simulink model "playback"  (R2016b)
settings: Solver=FixedStepDiscrete  StartTime=47  StopTime=49  FixedStep=sample_time  RelTol=1e-3
undefined symbols (not defined in the file or in its folder): A_kalman_sea_swing, A_lpf_dtau, B1_lpf_dtau, B2_lpf_dtau, B_kalman_sea_swing, C_kalman_sea_swing, control_start_time, Discrete, fdesignblkfcn, gcbh, initial_dx_estimate, k_sea_low, kalman_load_to_deflect_transmission, lateral_motor_efficiency, P0_kalman_sea_swing, Q_kalman_rotor_torque, Q_kalman_spring_torque, Q_kalman_trunk_torque, R_kalman_absolute_fail, R_kalman_absolute_normal, R_kalman_incremental_loaded, R_kalman_incremental_unloaded, sample_time, Time
libraries: simulink x4, ctrlSharedLib x4, dsparch4 x1
settings Model: Creator=wmartin  LastModifiedBy=Will
settings SolverCC: EnableConcurrentExecution=on
settings DataIOCC: MaxDataPoints=1000000000  SaveFormat=StructureWithTime  SignalLogging=off  DSMLogging=off  VisualizeSimOutput=off
settings OptimizationCC: BlockReduction=off  OptimizeBlockIOStorage=off  BufferReuse=off  GlobalBufferReuse=off  ExpressionFolding=off  ExpressionDepthLimit=2147483647  LocalBlockOutputs=off  LifeSpan=inf  SimCompilerOptimization=on
settings DebuggingCC: UnderspecifiedInitializationDetection=Classic  MergeDetectMultiDrivingBlocksExec=none  SolverPrmCheckMsg=warning  StateNameClashWarn=warning  SFUnexpectedBacktrackingDiag=warning  SFNoUnconditionalDefaultTransitionDiag=warning  SFExecutionAtInitializationDiag=none
settings HardwareCC: ProdBitPerPointer=32  ProdBitPerSizeT=32  ProdBitPerPtrDiffT=32  ProdLargestAtomicFloat=None  ProdWordSize=32  ProdLongLongMode=on  ProdHWDeviceType=Generic->32-bit x86 compatible
settings ModelReferenceCC: UpdateModelReferenceTargets=IfOutOfDate  ModelReferenceNumInstancesAllowed=Single  ModelReferenceMinAlgLoopOccurrences=on  PropagateSignalLabelsOutOfModel=off
settings RTWCC: SystemTargetFile=slrt.tlc  TemplateMakefile=slrt_default_tmf  Description=Simulink Real-Time  RTWVerbose=off  RTWCompilerOptimization=on
settings CodeAppCC: MaxIdLength=256
settings SimulinkRealTimeCC: GeneratePreprocessorConditionals=Disable all
settings ConfigComp: CovMetricSettings=dw  CovHtmlReporting=on  CovSaveCumulativeToWorkspaceVar=on  CovSaveSingleToWorkspaceVar=on  CovExternalEMLEnable=off  CovSFcnEnable=off

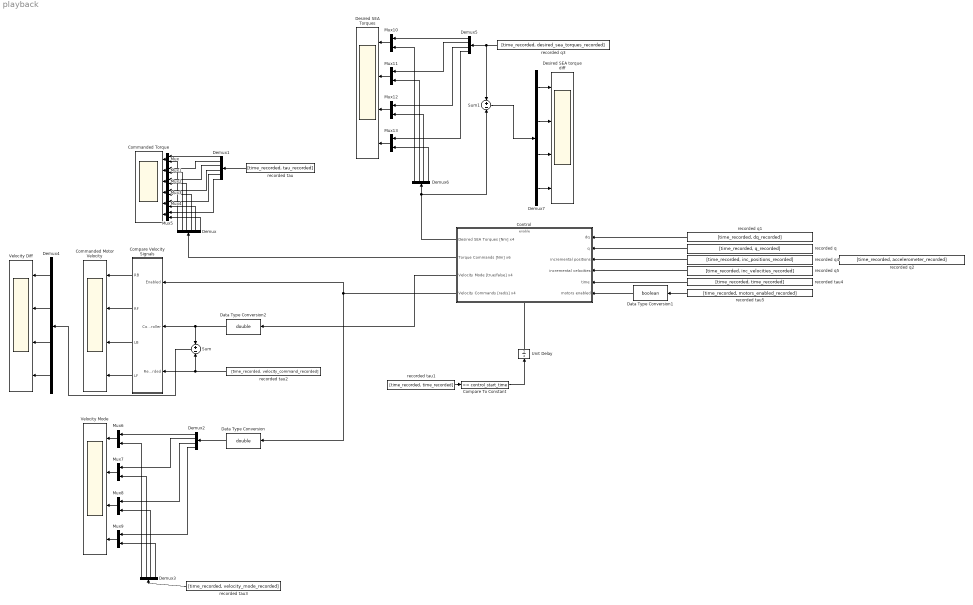
== system playback ==
  Commanded Motor Velocity : Scope  NumInputPorts=4
  Commanded Torque : Scope  NumInputPorts=6
  Compare To Constant : simulink/Logic and Bit Operations/Compare To Constant  relop=>=  const=control_start_time  OutDataTypeStr=boolean
  Compare Velocity Signals : Subsystem
  Control : Subsystem
  Data Type Conversion : DataTypeConversion  OutDataTypeStr=double
  Data Type Conversion1 : DataTypeConversion  OutDataTypeStr=boolean
  Data Type Conversion2 : DataTypeConversion  OutDataTypeStr=double
  Demux : Demux  Outputs=6
  Demux1 : Demux  Outputs=6
  Demux{2..7} (6 alike) : Demux
  Desired SEA Torques : Scope  NumInputPorts=4
  Desired SEA torque diff : Scope  NumInputPorts=4
  Mux{,1..13} (14 alike) : Mux  Inputs=2
  Sum : Sum  Inputs=+-
  Sum1 : Sum  Inputs=+-
  Unit Delay : UnitDelay  SampleTime=-1
  Velocity Diff : Scope  NumInputPorts=4
  Velocity Mode : Scope  NumInputPorts=4
  recorded q : FromWorkspace  VariableName=[time_recorded, q_recorded]  OutDataTypeStr=double  SampleTime=sample_time  OutputAfterFinalValue=Holding final value
  recorded q1 : FromWorkspace  VariableName=[time_recorded, dq_recorded]  OutDataTypeStr=double  SampleTime=sample_time  OutputAfterFinalValue=Holding final value
  recorded q2 : FromWorkspace  VariableName=[time_recorded, accelerometer_recorded]  OutDataTypeStr=double  SampleTime=sample_time  OutputAfterFinalValue=Holding final value
  recorded q3 : FromWorkspace  VariableName=[time_recorded, desired_sea_torques_recorded]  OutDataTypeStr=double  SampleTime=sample_time  OutputAfterFinalValue=Holding final value
  recorded q4 : FromWorkspace  VariableName=[time_recorded, inc_positions_recorded]  OutDataTypeStr=double  SampleTime=sample_time  OutputAfterFinalValue=Holding final value
  recorded q5 : FromWorkspace  VariableName=[time_recorded, inc_velocities_recorded]  OutDataTypeStr=double  SampleTime=sample_time  OutputAfterFinalValue=Holding final value
  recorded tau : FromWorkspace  VariableName=[time_recorded, tau_recorded]  OutDataTypeStr=double  SampleTime=sample_time  Interpolate=off  OutputAfterFinalValue=Holding final value
  recorded tau1 : FromWorkspace  VariableName=[time_recorded, time_recorded]  OutDataTypeStr=double  SampleTime=sample_time  OutputAfterFinalValue=Holding final value
  recorded tau2 : FromWorkspace  VariableName=[time_recorded, velocity_command_recorded]  OutDataTypeStr=double  SampleTime=sample_time  Interpolate=off  OutputAfterFinalValue=Holding final value
  recorded tau3 : FromWorkspace  VariableName=[time_recorded, velocity_mode_recorded]  OutDataTypeStr=double  SampleTime=sample_time  Interpolate=off  OutputAfterFinalValue=Holding final value
  recorded tau4 : FromWorkspace  VariableName=[time_recorded, time_recorded]  OutDataTypeStr=double  SampleTime=sample_time  OutputAfterFinalValue=Holding final value
  recorded tau5 : FromWorkspace  VariableName=[time_recorded, motors_enabled_recorded]  OutDataTypeStr=double  SampleTime=sample_time  OutputAfterFinalValue=Holding final value
  wires:
  recorded tau1/1 -> Compare To Constant/1
  Compare To Constant/1 -> Unit Delay/1
  Unit Delay/1 -> Control/Enable
  Control/2(Torque Commands [Nm] x6) -> Demux/1
  recorded tau/1 -> Demux1/1
  Mux/1 -> Commanded Torque/1
  Mux1/1 -> Commanded Torque/2
  Mux2/1 -> Commanded Torque/3
  Mux3/1 -> Commanded Torque/4
  Mux4/1 -> Commanded Torque/5
  Mux5/1 -> Commanded Torque/6
  Demux1/1 -> Mux/1
  Demux/1 -> Mux/2
  Demux1/2 -> Mux1/1
  Demux1/3 -> Mux2/1
  Demux1/4 -> Mux3/1
  Demux1/5 -> Mux4/1
  Demux1/6 -> Mux5/1
  Demux/2 -> Mux1/2
  Demux/3 -> Mux2/2
  Demux/4 -> Mux3/2
  Demux/5 -> Mux4/2
  Demux/6 -> Mux5/2
  Compare Velocity Signals/1(RB) -> Commanded Motor Velocity/1
  Compare Velocity Signals/2(RF) -> Commanded Motor Velocity/2
  Compare Velocity Signals/3(LB) -> Commanded Motor Velocity/3
  Compare Velocity Signals/4(LF) -> Commanded Motor Velocity/4
  Control/4(Velocity Commands [rad/s] x4) -> Compare Velocity Signals/1(Enabled), Data Type Conversion/1
  recorded tau2/1 -> Sum/2, Compare Velocity Signals/3(Recorded)
  Mux6/1 -> Velocity Mode/1
  Mux7/1 -> Velocity Mode/2
  Mux8/1 -> Velocity Mode/3
  Mux9/1 -> Velocity Mode/4
  Demux2/2 -> Mux7/1
  Demux2/3 -> Mux8/1
  Demux2/4 -> Mux9/1
  recorded tau3/1 -> Demux3/1
  Demux3/1 -> Mux6/2
  Demux3/2 -> Mux7/2
  Demux3/3 -> Mux8/2
  Demux3/4 -> Mux9/2
  Data Type Conversion/1 -> Demux2/1
  Demux2/1 -> Mux6/1
  Control/3(Velocity Mode [true/false] x4) -> Data Type Conversion2/1
  Sum/1 -> Demux4/1
  Demux4/4 -> Velocity Diff/4
  Demux4/3 -> Velocity Diff/3
  Demux4/2 -> Velocity Diff/2
  Demux4/1 -> Velocity Diff/1
  Mux10/1 -> Desired SEA Torques/1
  Mux11/1 -> Desired SEA Torques/2
  Mux12/1 -> Desired SEA Torques/3
  Mux13/1 -> Desired SEA Torques/4
  Demux5/2 -> Mux11/1
  Demux5/3 -> Mux12/1
  Demux5/4 -> Mux13/1
  Demux6/1 -> Mux10/2
  Demux6/2 -> Mux11/2
  Demux6/3 -> Mux12/2
  Demux6/4 -> Mux13/2
  recorded q3/1 -> Demux5/1, Sum1/1
  Demux5/1 -> Mux10/1
  Control/1(Desired SEA Torques [Nm] x4) -> Sum1/2, Demux6/1
  Demux7/3 -> Desired SEA torque diff/3
  Demux7/2 -> Desired SEA torque diff/2
  Demux7/1 -> Desired SEA torque diff/1
  Demux7/4 -> Desired SEA torque diff/4
  Sum1/1 -> Demux7/1
  recorded q1/1 -> Control/1(dq)
  recorded q/1 -> Control/2(q)
  recorded tau4/1 -> Control/5(time)
  Data Type Conversion1/1 -> Control/6(motors enabled)
  recorded tau5/1 -> Data Type Conversion1/1
  recorded q4/1 -> Control/3(incremental positions)
  recorded q5/1 -> Control/4(incremental velocities)
  Data Type Conversion2/1 -> Sum/1, Compare Velocity Signals/2(Controller)

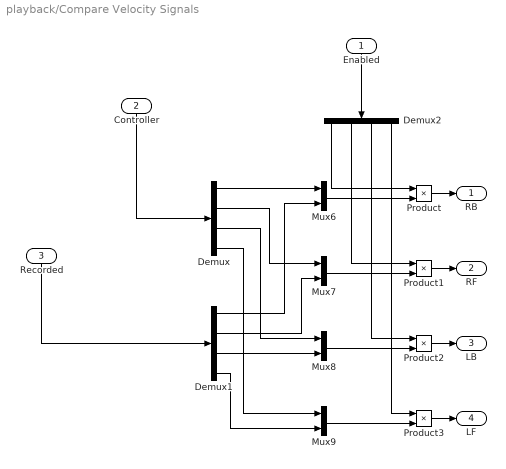
== system playback/Compare Velocity Signals ==
  Enabled : Inport
  Controller : Inport  Port=2
  Recorded : Inport  Port=3
  Demux : Demux
  Demux1 : Demux
  Demux2 : Demux
  Mux{6..9} (4 alike) : Mux  Inputs=2
  Product{,1..3} (4 alike) : Product
  RB : Outport
  RF : Outport  Port=2
  LB : Outport  Port=3
  LF : Outport  Port=4
  wires:
  Demux/3 -> Mux8/1
  Demux/2 -> Mux7/1
  Demux1/1 -> Mux6/2
  Demux/1 -> Mux6/1
  Product/1 -> RB/1
  Demux/4 -> Mux9/1
  Mux6/1 -> Product/2
  Demux1/4 -> Mux9/2
  Mux7/1 -> Product1/2
  Mux9/1 -> Product3/2
  Recorded/1 -> Demux1/1
  Demux2/3 -> Product2/1
  Demux1/2 -> Mux7/2
  Controller/1 -> Demux/1
  Demux2/1 -> Product/1
  Product3/1 -> LF/1
  Product1/1 -> RF/1
  Product2/1 -> LB/1
  Mux8/1 -> Product2/2
  Demux1/3 -> Mux8/2
  Enabled/1 -> Demux2/1
  Demux2/4 -> Product3/1
  Demux2/2 -> Product1/1

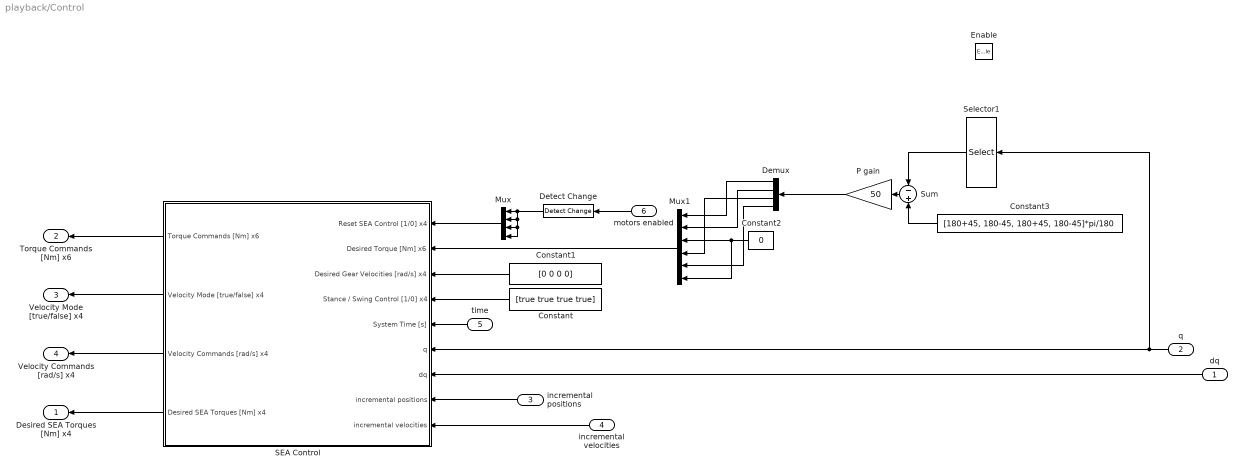
== system playback/Control ==
  dq : Inport
  q : Inport  Port=2
  incremental positions : Inport  Port=3
  incremental velocities : Inport  Port=4
  time : Inport  Port=5
  motors enabled : Inport  Port=6
  Enable : EnablePort  StatesWhenEnabling=reset  PropagateVarSize=During execution  ShowOutputPort=on
  Constant : Constant  Value=[true true true true]
  Constant1 : Constant  Value=[0 0 0 0]
  Constant2 : Constant  Value=0
  Constant3 : Constant  Value=[180+45, 180-45, 180+45, 180-45]*pi/180
  Demux : Demux
  Detect Change : simulink/Logic and Bit Operations/Detect Change  vinit=0  InputProcessing=Inherited  OutDataTypeStr=boolean
  Mux : Mux
  Mux1 : Mux  Inputs=6
  P gain : Gain  Gain=50
  SEA Control : Subsystem
  Selector1 : Selector  InputPortWidth=13  IndexOptions=Index vector (dialog)  Indices=[1 3 5 7]  OutputSizes=1
  Sum : Sum  Inputs=-+
  Desired SEA Torques [Nm] x4 : Outport  InitialOutput=[0 0 0 0]
  Torque Commands [Nm] x6 : Outport  Port=2  InitialOutput=[0 0 0 0 0 0]
  Velocity Mode [true/false] x4 : Outport  Port=3  InitialOutput=[false false false false]
  Velocity Commands [rad/s] x4 : Outport  Port=4  InitialOutput=[0 0 0 0]
  wires:
  incremental velocities/1 -> SEA Control/9(incremental velocities)
  incremental positions/1 -> SEA Control/8(incremental positions)
  P gain/1 -> Demux/1
  Sum/1 -> P gain/1
  Constant3/1 -> Sum/2
  Selector1/1 -> Sum/1
  Demux/4 -> Mux1/5
  Demux/3 -> Mux1/4
  Demux/2 -> Mux1/2
  Demux/1 -> Mux1/1
  Constant2/1 -> Mux1/3, Mux1/6
  SEA Control/4(Desired SEA Torques [Nm] x4) -> Desired SEA Torques [Nm] x4/1
  SEA Control/3(Velocity Commands [rad/s] x4) -> Velocity Commands [rad/s] x4/1
  SEA Control/2(Velocity Mode [true/false] x4) -> Velocity Mode [true/false] x4/1
  SEA Control/1(Torque Commands [Nm] x6) -> Torque Commands [Nm] x6/1
  Constant/1 -> SEA Control/4(Stance / Swing Control [1/0] x4)
  Constant1/1 -> SEA Control/3(Desired Gear Velocities [rad/s] x4)
  Mux1/1 -> SEA Control/2(Desired Torque [Nm] x6)
  Mux/1 -> SEA Control/1(Reset SEA Control [1/0] x4)
  dq/1 -> SEA Control/7(dq)
  q/1 -> Selector1/1, SEA Control/6(q)
  motors enabled/1 -> Detect Change/1
  Detect Change/1 -> Mux/4, Mux/3, Mux/2, Mux/1
  time/1 -> SEA Control/5(System Time [s])

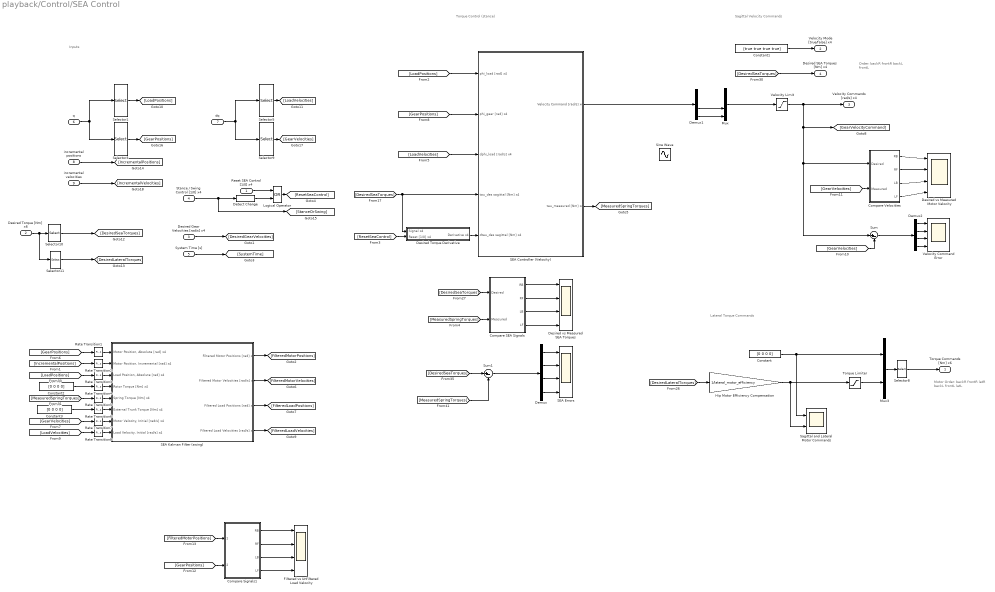
== system playback/Control/SEA Control ==
  note: Sagittal Velocity Commands
  note: Lateral Torque Commands
  note: Inputs
  note: Torque Control (stance)
  note: Motor Order:
      |
      | backR
      | frontR
      | latR
      | backL
      | frontL
      | latL
  note: Order:
      | backR
      | frontR
      | backL
      | frontL
  Reset SEA Control [1/0] x4 : Inport  OutDataTypeStr=boolean  PortDimensions=4  SampleTime=sample_time
  Desired Torque [Nm] x6 : Inport  Port=2  OutDataTypeStr=double  PortDimensions=6  SampleTime=sample_time
  Desired Gear Velocities [rad/s] x4 : Inport  Port=3  OutDataTypeStr=double  PortDimensions=4  SampleTime=sample_time
  Stance / Swing Control [1/0] x4 : Inport  Port=4  OutDataTypeStr=boolean  PortDimensions=4  SampleTime=sample_time
  System Time [s] : Inport  Port=5  OutDataTypeStr=double  PortDimensions=1  SampleTime=sample_time
  q : Inport  Port=6  OutDataTypeStr=double  PortDimensions=13  SampleTime=sample_time
  dq : Inport  Port=7  OutDataTypeStr=double  PortDimensions=13  SampleTime=sample_time
  incremental positions : Inport  Port=8  OutDataTypeStr=double  PortDimensions=4  SampleTime=sample_time
  incremental velocities : Inport  Port=9  OutDataTypeStr=double  PortDimensions=4  SampleTime=sample_time
  Compare SEA Signals : Subsystem
  Compare Signals1 : Subsystem
  Compare Velocities : Subsystem
  Constant : Constant  Value=[0 0 0 0]
  Constant1 : Constant  Value=[true true true true]
  Constant2 : Constant  Value=[0 0 0 0]
  Constant3 : Constant  Value=[0 0 0 0]
  Demux : Demux
  Demux1 : Demux
  Demux2 : Demux
  Desired Torque Derivative : Subsystem
  Desired vs Measured Motor Velocity : Scope  NumInputPorts=4
  Desired vs Measured SEA Torques : Scope  NumInputPorts=4
  Detect Change : simulink/Logic and Bit Operations/Detect Change  vinit=0  InputProcessing=Inherited  OutDataTypeStr=boolean
  Filtered vs Unfiltered Load Velocity : Scope  NumInputPorts=4
  Hip Motor Efficiency Compensation : Gain  Gain=1/lateral_motor_efficiency
  Logical Operator : Logic  Operator=OR  AllPortsSameDT=off  OutDataTypeStr=boolean
  Mux : Mux
  Mux3 : Mux  Inputs=2
  Rate Transition{1..8} (8 alike) : RateTransition  OutPortSampleTime=sample_time
  SEA Controller (Velocity) : Subsystem
  SEA Errors : Scope  NumInputPorts=4
  SEA Kalman Filter (swing) : Subsystem
  Sagittal and Lateral Motor Commands : Scope  NumInputPorts=2
  Selector1 : Selector  InputPortWidth=13  IndexOptions=Index vector (dialog)  Indices=[1 3 5 7]  OutputSizes=1
  Selector10 : Selector  InputPortWidth=6  IndexOptions=Index vector (dialog)  Indices=[1 2 4 5]  OutputSizes=1
  Selector11 : Selector  InputPortWidth=6  IndexOptions=Index vector (dialog)  Indices=[3 6]  OutputSizes=1
  Selector3 : Selector  InputPortWidth=13  IndexOptions=Index vector (dialog)  Indices=[2 4 6 8]  OutputSizes=1
  Selector5 : Selector  InputPortWidth=13  IndexOptions=Index vector (dialog)  Indices=[1 3 5 7]  OutputSizes=1
  Selector8 : Selector  InputPortWidth=6  IndexOptions=Index vector (dialog)  Indices=[1 2 5 3 4 6]  OutputSizes=1
  Selector9 : Selector  InputPortWidth=13  IndexOptions=Index vector (dialog)  Indices=[2 4 6 8]  OutputSizes=1
  Sine Wave : Sin  Amplitude=0.2  Frequency=68*2*pi  SampleTime=sample_time
  Sum : Sum  Inputs=|+-
  Sum1 : Sum  Inputs=|+-
  Torque Limiter : Saturate  UpperLimit=200  LowerLimit=-200
      settings: AttributesFormatString=Hi: %<UpperLimit>\nLo: %<LowerLimit>
  Velocity Command Error : Scope  NumInputPorts=4
  Velocity Limit : Saturate  UpperLimit=6  LowerLimit=-6
      settings: AttributesFormatString=Hi: %<UpperLimit>\nLo: %<LowerLimit>
  Torque Commands [Nm] x6 : Outport  OutDataTypeStr=double  PortDimensions=6  SampleTime=sample_time  InitialOutput=[0 0 0 0 0 0]
  Velocity Mode [true/false] x4 : Outport  Port=2  InitialOutput=[false false false false]
  Velocity Commands [rad/s] x4 : Outport  Port=3  InitialOutput=[0 0 0 0]
  Desired SEA Torques [Nm] x4 : Outport  Port=4  InitialOutput=[false false false false]
  wires:
  SEA Kalman Filter (swing)/4(Filtered Load Velocities [rad/s] x4) -> [FilteredLoadVelocities]
  SEA Kalman Filter (swing)/2(Filtered Motor Velocities [rad/s] x4) -> [FilteredMotorVelocities]
  SEA Kalman Filter (swing)/3(Filtered Load Positions [rad] x4) -> [FilteredLoadPositions]
  SEA Kalman Filter (swing)/1(Filtered Motor Positions [rad] x4) -> [FilteredMotorPositions]
  Constant3/1 -> Rate Transition6/1
  [LoadVelocities] -> Rate Transition8/1
  [GearVelocities] -> Rate Transition7/1
  Constant2/1 -> Rate Transition4/1
  [IncrementalPositions] -> Rate Transition2/1
  [GearPositions] -> Rate Transition1/1
  [LoadPositions] -> Rate Transition3/1
  [MeasuredSpringTorques] -> Rate Transition5/1
  incremental velocities/1 -> [IncrementalVelocities]
  incremental positions/1 -> [IncrementalPositions]
  Demux1/3 -> Mux/3
  Demux1/4 -> Mux/4
  Mux/1 -> Velocity Limit/1
  Torque Limiter/1 -> Mux3/2
  Sum1/1 -> Demux/1
  Demux/2 -> SEA Errors/2
  Demux/3 -> SEA Errors/3
  Demux/4 -> SEA Errors/4
  Demux/1 -> SEA Errors/1
  [DesiredSeaTorques] -> Sum1/1
  [MeasuredSpringTorques] -> Sum1/2
  Velocity Limit/1 -> Velocity Commands [rad/s] x4/1, Compare Velocities/1(Desired), Sum/1, [GearVelocityCommand]
  System Time [s]/1 -> [SystemTime]
  Selector9/1 -> [GearVelocities]
  Desired Gear Velocities [rad/s] x4/1 -> [DesiredGearVelocities]
  Detect Change/1 -> Logical Operator/2
  SEA Controller (Velocity)/1(Velocity Command [rad/s] x4) -> Demux1/1
  Selector10/1 -> [DesiredSeaTorques]
  Demux2/1 -> Velocity Command Error/1
  Demux2/2 -> Velocity Command Error/2
  Demux2/3 -> Velocity Command Error/3
  Demux2/4 -> Velocity Command Error/4
  Sum/1 -> Demux2/1
  [GearVelocities] -> Sum/2
  [GearVelocities] -> Compare Velocities/2(Measured)
  [GearPositions] -> SEA Controller (Velocity)/2(phi_gear [rad] x4)
  dq/1 -> Selector9/1, Selector5/1
  Selector3/1 -> [GearPositions]
  [LoadVelocities] -> SEA Controller (Velocity)/3(dphi_load [rad/s] x4)
  [DesiredSeaTorques] -> Desired SEA Torques [Nm] x4/1
  Reset SEA Control [1/0] x4/1 -> Logical Operator/1
  Logical Operator/1 -> [ResetSeaControl]
  Stance / Swing Control [1/0] x4/1 -> Detect Change/1, [StanceOrSwing]
  Constant1/1 -> Velocity Mode [true/false] x4/1
  [ResetSeaControl] -> Desired Torque Derivative/2(Reset [1/0] x4)
  [DesiredSeaTorques] -> Compare SEA Signals/1(Desired)
  Selector11/1 -> [DesiredLateralTorques]
  Desired Torque [Nm] x6/1 -> Selector10/1, Selector11/1
  Selector5/1 -> [LoadVelocities]
  Selector1/1 -> [LoadPositions]
  [MeasuredSpringTorques] -> Compare SEA Signals/2(Measured)
  Compare Velocities/2(RF) -> Desired vs Measured Motor Velocity/2
  Compare Velocities/1(RB) -> Desired vs Measured Motor Velocity/1
  Compare Velocities/3(LB) -> Desired vs Measured Motor Velocity/3
  Compare Velocities/4(LF) -> Desired vs Measured Motor Velocity/4
  Compare SEA Signals/4(LF) -> Desired vs Measured SEA Torques/4
  Compare SEA Signals/3(LB) -> Desired vs Measured SEA Torques/3
  Compare SEA Signals/2(RF) -> Desired vs Measured SEA Torques/2
  Compare SEA Signals/1(RB) -> Desired vs Measured SEA Torques/1
  Hip Motor Efficiency Compensation/1 -> Torque Limiter/1, Sagittal and Lateral Motor Commands/2
  Constant/1 -> Mux3/1, Sagittal and Lateral Motor Commands/1
  Desired Torque Derivative/1(Derivative x4) -> SEA Controller (Velocity)/5(dtau_des sagittal [Nm] x4)
  Mux3/1 -> Selector8/1
  [DesiredLateralTorques] -> Hip Motor Efficiency Compensation/1
  [DesiredSeaTorques] -> SEA Controller (Velocity)/4(tau_des sagittal [Nm] x4), Desired Torque Derivative/1(Signal x4)
  [LoadPositions] -> SEA Controller (Velocity)/1(phi_load [rad] x4)
  q/1 -> Selector3/1, Selector1/1
  Selector8/1 -> Torque Commands [Nm] x6/1
  SEA Controller (Velocity)/2(tau_measured [Nm] x4) -> [MeasuredSpringTorques]
  Compare Signals1/4(LF) -> Filtered vs Unfiltered Load Velocity/4
  Compare Signals1/3(LB) -> Filtered vs Unfiltered Load Velocity/3
  Compare Signals1/2(RF) -> Filtered vs Unfiltered Load Velocity/2
  Compare Signals1/1(RB) -> Filtered vs Unfiltered Load Velocity/1
  [GearPositions] -> Compare Signals1/2(2)
  [FilteredMotorPositions] -> Compare Signals1/1(1)
  Rate Transition1/1 -> SEA Kalman Filter (swing)/1("Motor Position, Absolute [rad] x4")
  Rate Transition2/1 -> SEA Kalman Filter (swing)/2("Motor Position, Incremental [rad] x4")
  Rate Transition3/1 -> SEA Kalman Filter (swing)/3("Load Position, Absolute [rad] x4")
  Rate Transition4/1 -> SEA Kalman Filter (swing)/4(Rotor Torque [Nm] x4)
  Rate Transition5/1 -> SEA Kalman Filter (swing)/5(Spring Torque [Nm] x4)
  Rate Transition6/1 -> SEA Kalman Filter (swing)/6(External Trunk Torque [Nm] x4)
  Rate Transition7/1 -> SEA Kalman Filter (swing)/7("Motor Velocity, Initial [rad/s] x4")
  Rate Transition8/1 -> SEA Kalman Filter (swing)/8("Load Velocity, Initial [rad/s] x4")

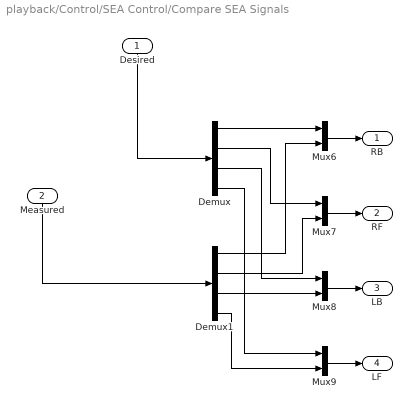
== system playback/Control/SEA Control/Compare SEA Signals ==
  Desired : Inport
  Measured : Inport  Port=2
  Demux : Demux
  Demux1 : Demux
  Mux{6..9} (4 alike) : Mux  Inputs=2
  RB : Outport
  RF : Outport  Port=2
  LB : Outport  Port=3
  LF : Outport  Port=4
  wires:
  Mux8/1 -> LB/1
  Mux9/1 -> LF/1
  Mux7/1 -> RF/1
  Mux6/1 -> RB/1
  Demux1/3 -> Mux8/2
  Desired/1 -> Demux/1
  Demux1/2 -> Mux7/2
  Measured/1 -> Demux1/1
  Demux1/4 -> Mux9/2
  Demux/4 -> Mux9/1
  Demux/1 -> Mux6/1
  Demux1/1 -> Mux6/2
  Demux/2 -> Mux7/1
  Demux/3 -> Mux8/1

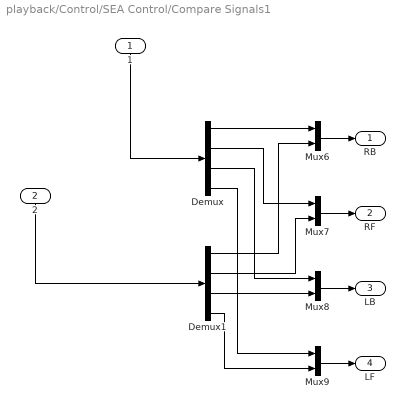
== system playback/Control/SEA Control/Compare Signals1 ==
  1 : Inport
  2 : Inport  Port=2
  Demux : Demux
  Demux1 : Demux
  Mux{6..9} (4 alike) : Mux  Inputs=2
  RB : Outport
  RF : Outport  Port=2
  LB : Outport  Port=3
  LF : Outport  Port=4
  wires:
  Demux/3 -> Mux8/1
  Demux/2 -> Mux7/1
  Demux1/1 -> Mux6/2
  Demux/1 -> Mux6/1
  Demux/4 -> Mux9/1
  Demux1/4 -> Mux9/2
  2/1 -> Demux1/1
  Demux1/2 -> Mux7/2
  1/1 -> Demux/1
  Demux1/3 -> Mux8/2
  Mux6/1 -> RB/1
  Mux7/1 -> RF/1
  Mux9/1 -> LF/1
  Mux8/1 -> LB/1

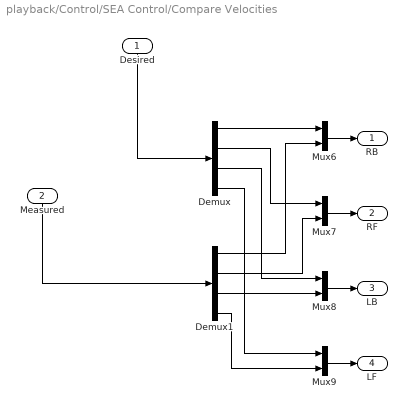
== system playback/Control/SEA Control/Compare Velocities ==
  Desired : Inport
  Measured : Inport  Port=2
  Demux : Demux
  Demux1 : Demux
  Mux{6..9} (4 alike) : Mux  Inputs=2
  RB : Outport
  RF : Outport  Port=2
  LB : Outport  Port=3
  LF : Outport  Port=4
  wires:
  Mux9/1 -> LF/1
  Mux8/1 -> LB/1
  Mux7/1 -> RF/1
  Mux6/1 -> RB/1
  Demux/3 -> Mux8/1
  Demux/2 -> Mux7/1
  Demux1/1 -> Mux6/2
  Demux/1 -> Mux6/1
  Demux/4 -> Mux9/1
  Demux1/4 -> Mux9/2
  Measured/1 -> Demux1/1
  Demux1/2 -> Mux7/2
  Desired/1 -> Demux/1
  Demux1/3 -> Mux8/2

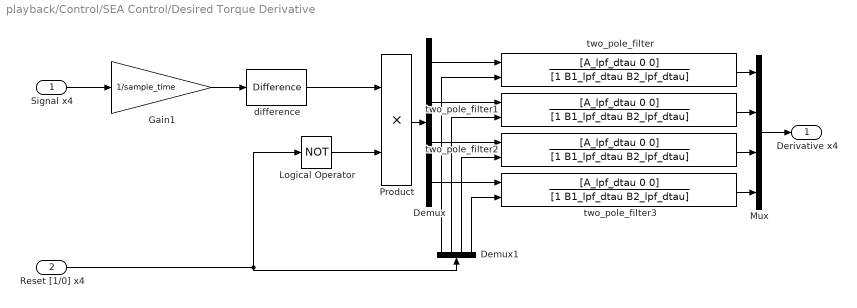
== system playback/Control/SEA Control/Desired Torque Derivative ==
  Signal x4 : Inport
  Reset [1/0] x4 : Inport  Port=2
  Demux : Demux
  Demux1 : Demux
  Gain1 : Gain  Gain=1/sample_time
  Logical Operator : Logic  Operator=NOT  AllPortsSameDT=off  OutDataTypeStr=boolean
  Mux : Mux
  Product : Product
  difference : simulink/Discrete/Difference  ICPrevInput=0.0  InputProcessing=Inherited  OutMin=[]  OutMax=[]  OutDataType=fixdt(1, 16)  OutScaling=2^-10  DoSatur=off
  two_pole_filter{,1..3} (4 alike) : DiscreteTransferFcn  Numerator=[A_lpf_dtau 0 0]  Denominator=[1 B1_lpf_dtau B2_lpf_dtau]  ExternalReset=Rising  SampleTime=sample_time
      settings: InputPortMap=u0,r7
  Derivative x4 : Outport
  wires:
  Demux1/4 -> two_pole_filter3/2
  Demux1/3 -> two_pole_filter2/2
  Demux1/2 -> two_pole_filter1/2
  Demux1/1 -> two_pole_filter/2
  Demux/4 -> two_pole_filter3/1
  Demux/3 -> two_pole_filter2/1
  Demux/2 -> two_pole_filter1/1
  two_pole_filter3/1 -> Mux/4
  two_pole_filter2/1 -> Mux/3
  two_pole_filter1/1 -> Mux/2
  Product/1 -> Demux/1
  two_pole_filter/1 -> Mux/1
  Reset [1/0] x4/1 -> Logical Operator/1, Demux1/1
  Logical Operator/1 -> Product/2
  Gain1/1 -> difference/1
  Signal x4/1 -> Gain1/1
  Mux/1 -> Derivative x4/1
  difference/1 -> Product/1
  Demux/1 -> two_pole_filter/1

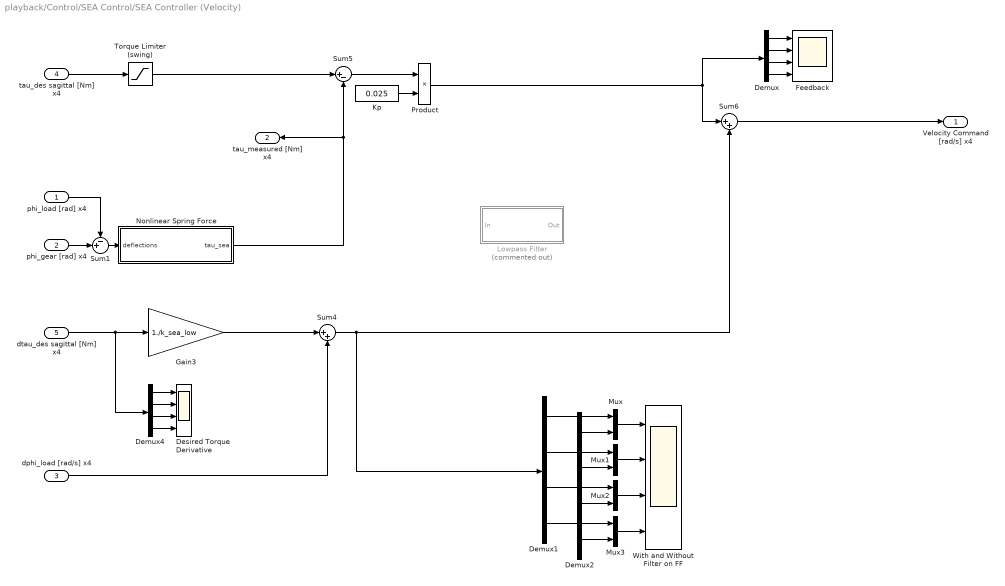
== system playback/Control/SEA Control/SEA Controller (Velocity) ==
  phi_load [rad] x4 : Inport
  phi_gear [rad] x4 : Inport  Port=2
  dphi_load [rad/s] x4 : Inport  Port=3
  tau_des sagittal [Nm] x4 : Inport  Port=4
  dtau_des sagittal [Nm] x4 : Inport  Port=5
  Demux{,1..2,4} (4 alike) : Demux
  Desired Torque Derivative : Scope  NumInputPorts=4
  Feedback : Scope  NumInputPorts=4
  Gain3 : Gain  Gain=1./k_sea_low
  Kp : Constant  Value=0.025
  Lowpass Filter : Subsystem  Commented=on  DialogController=fdesignblkfcn  InitFcn=fdesignblkfcn(gcbh, {'InitFcn'});  mask(Lowpass Filter){}
      mask help: Design a lowpass filter
      settings: CopyFcn=fdesignblkfcn(gcbh, {'CopyFcn'});
      mask Help: helpview(mapfilelocation('dsp'), 'dsplowpassfilter');
      mask Display: disp('Lowpass')
  Mux{,1..3} (4 alike) : Mux  Inputs=2
  Nonlinear Spring Force : MATLAB Function  TreatAsAtomicUnit=on
  Product : Product
  Sum1 : Sum  Inputs=-+|
  Sum4 : Sum  Inputs=|++
  Sum5 : Sum  Inputs=|+-
  Sum6 : Sum  Inputs=|++
  Torque Limiter (swing) : Saturate  UpperLimit=80  LowerLimit=-80
      settings: AttributesFormatString=Hi: %<UpperLimit>\nLo: %<LowerLimit>
  With and Without Filter on FF : Scope  NumInputPorts=4
  Velocity Command [rad/s] x4 : Outport  PortDimensions=4
  tau_measured [Nm] x4 : Outport  Port=2
  wires:
  Sum4/1 -> Demux1/1, Sum6/2
  Demux2/1 -> Mux/2
  Demux2/2 -> Mux1/2
  Demux2/3 -> Mux2/2
  Demux2/4 -> Mux3/2
  Demux1/4 -> Mux3/1
  Demux1/3 -> Mux2/1
  Demux1/2 -> Mux1/1
  Demux1/1 -> Mux/1
  Mux3/1 -> With and Without Filter on FF/4
  Mux2/1 -> With and Without Filter on FF/3
  Mux1/1 -> With and Without Filter on FF/2
  Mux/1 -> With and Without Filter on FF/1
  Sum6/1 -> Velocity Command [rad/s] x4/1
  Product/1 -> Demux/1, Sum6/1
  Demux4/1 -> Desired Torque Derivative/1
  Demux4/2 -> Desired Torque Derivative/2
  Demux4/3 -> Desired Torque Derivative/3
  Demux4/4 -> Desired Torque Derivative/4
  phi_load [rad] x4/1 -> Sum1/1
  phi_gear [rad] x4/1 -> Sum1/2
  tau_des sagittal [Nm] x4/1 -> Torque Limiter (swing)/1
  Demux/1 -> Feedback/1
  Demux/2 -> Feedback/2
  Demux/3 -> Feedback/3
  Demux/4 -> Feedback/4
  Torque Limiter (swing)/1 -> Sum5/1
  Kp/1 -> Product/2
  dphi_load [rad/s] x4/1 -> Sum4/2
  Sum5/1 -> Product/1
  dtau_des sagittal [Nm] x4/1 -> Gain3/1, Demux4/1
  Gain3/1 -> Sum4/1
  Nonlinear Spring Force/1(tau_sea) -> Sum5/2, tau_measured [Nm] x4/1
  Sum1/1 -> Nonlinear Spring Force/1(deflections)

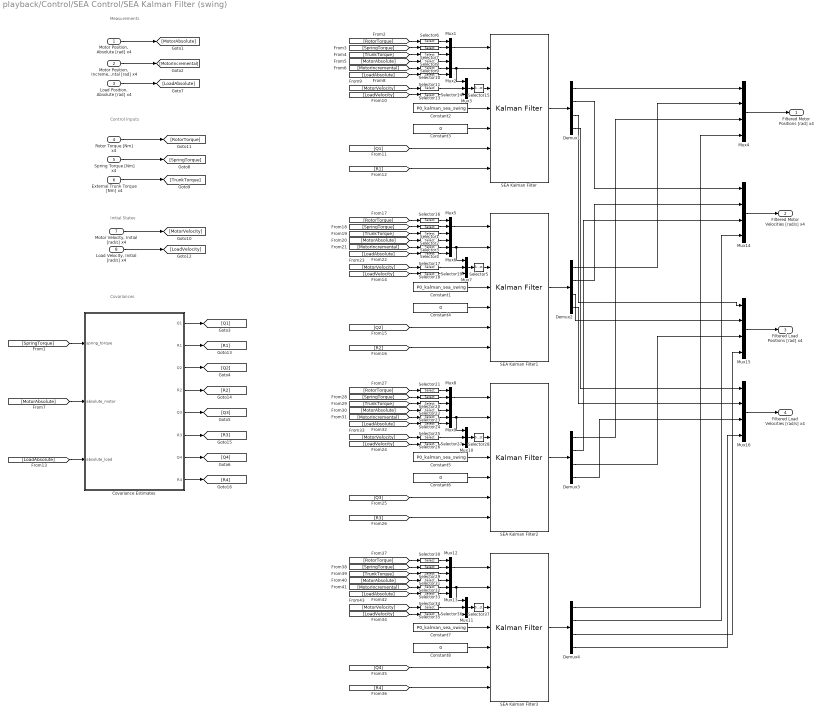
== system playback/Control/SEA Control/SEA Kalman Filter (swing) ==
  note: Covariances
  note: Initial States
  note: Control Inputs
  note: Measurements
  "Motor Position, Absolute [rad] x4" : Inport
  "Motor Position, Incremental [rad] x4" : Inport  Port=2
  "Load Position, Absolute [rad] x4" : Inport  Port=3
  Rotor Torque [Nm] x4 : Inport  Port=4
  Spring Torque [Nm] x4 : Inport  Port=5
  External Trunk Torque [Nm] x4 : Inport  Port=6
  "Motor Velocity, Initial [rad/s] x4" : Inport  Port=7
  "Load Velocity, Initial [rad/s] x4" : Inport  Port=8
  Constant{1..2,5,7} (4 alike) : Constant  Value=P0_kalman_sea_swing
  Constant{3..4,6,8} (4 alike) : Constant  Value=0
  Covariance Estimates : MATLAB Function  TreatAsAtomicUnit=on
  Demux{1..4} (4 alike) : Demux
  Mux{1..3,5..13} (12 alike) : Mux  Inputs=3
  Mux{4,14..16} (4 alike) : Mux
  SEA Kalman Filter{,1..3} (4 alike) : ctrlSharedLib/Kalman Filter  TimeDomain=Discrete-Time  UseCurrentEstimator=on  ModelSource=Individual A, B, C, D matrices  ModelSourceVariable=A_kf  A=A_kalman_sea_swing  B=B_kalman_sea_swing  C=C_kalman_sea_swing  D=0  NumberOfStates=2  NumberOfInputs=1  NumberOfOutputs=2  InitialEstimateSource=Input port  X0=initial_dx_estimate  P0=P0_kalman_transverse  UseK=off  UseGH=on  NumberOfProcessNoiseInputs=1  G=G_kalman_sea_swing  TimeInvariantG=on  H=0  TimeInvariantH=on  Q=1  TimeInvariantQ=off  R=1  TimeInvariantR=off  N=0  TimeInvariantN=on  AddInputPort=on  AddEnablePort=off  ExternalReset=Rising  OutputEstimatedY=off  OutputP=off  Ts=sample_time
  Selector{1..4,16..19} (8 alike) : Selector  InputPortWidth=4  IndexOptions=Index vector (dialog)  Indices=[2]  OutputSizes=1
  Selector{6..11,13..14} (8 alike) : Selector  InputPortWidth=4  IndexOptions=Index vector (dialog)  Indices=[1]  OutputSizes=1
  Selector{5,15,28,37} (4 alike) : Selector  InputPortWidth=5  IndexOptions=Index vector (dialog)  Indices=[1 4 3 5]  OutputSizes=1
  Selector{20..27} (8 alike) : Selector  InputPortWidth=4  IndexOptions=Index vector (dialog)  Indices=[3]  OutputSizes=1
  Selector{29..36} (8 alike) : Selector  InputPortWidth=4  IndexOptions=Index vector (dialog)  Indices=[4]  OutputSizes=1
  Filtered Motor Positions [rad] x4 : Outport
  Filtered Motor Velocities [rad/s] x4 : Outport  Port=2
  Filtered Load Positions [rad] x4 : Outport  Port=3
  Filtered Load Velocities [rad/s] x4 : Outport  Port=4
  wires:
  [MotorAbsolute] -> Covariance Estimates/2(absolute_motor)
  [LoadAbsolute] -> Covariance Estimates/3(absolute_load)
  Demux4/4 -> Mux16/4
  Demux3/4 -> Mux16/3
  Demux2/4 -> Mux16/2
  Demux1/4 -> Mux16/1
  Demux4/3 -> Mux15/4
  Demux3/3 -> Mux15/3
  Demux2/3 -> Mux15/2
  Demux1/3 -> Mux15/1
  Demux4/2 -> Mux14/4
  Demux3/2 -> Mux14/3
  Demux2/2 -> Mux14/2
  Demux1/2 -> Mux14/1
  Demux4/1 -> Mux4/4
  Demux3/1 -> Mux4/3
  Demux2/1 -> Mux4/2
  Demux1/1 -> Mux4/1
  Mux16/1 -> Filtered Load Velocities [rad/s] x4/1
  Mux14/1 -> Filtered Motor Velocities [rad/s] x4/1
  Mux15/1 -> Filtered Load Positions [rad] x4/1
  SEA Kalman Filter3/1 -> Demux4/1
  [Q4] -> SEA Kalman Filter3/6
  [R4] -> SEA Kalman Filter3/7
  Constant8/1 -> SEA Kalman Filter3/5
  Constant7/1 -> SEA Kalman Filter3/4
  Selector37/1 -> SEA Kalman Filter3/3
  Selector35/1 -> Mux11/2
  Selector36/1 -> Mux11/3
  [LoadVelocity] -> Selector36/1
  [MotorVelocity] -> Selector35/1
  Mux11/1 -> Selector37/1
  [LoadAbsolute] -> Selector34/1
  [MotorIncremental] -> Selector33/1
  [MotorAbsolute] -> Selector32/1
  Selector32/1 -> Mux13/1
  Selector33/1 -> Mux13/2
  Selector34/1 -> Mux13/3
  [TrunkTorque] -> Selector31/1
  [SpringTorque] -> Selector29/1
  Selector31/1 -> Mux12/3
  Selector29/1 -> Mux12/2
  [RotorTorque] -> Selector30/1
  Selector30/1 -> Mux12/1
  Mux13/1 -> Mux11/1, SEA Kalman Filter3/2
  Mux12/1 -> SEA Kalman Filter3/1
  SEA Kalman Filter2/1 -> Demux3/1
  [Q3] -> SEA Kalman Filter2/6
  [R3] -> SEA Kalman Filter2/7
  Constant6/1 -> SEA Kalman Filter2/5
  Constant5/1 -> SEA Kalman Filter2/4
  Selector28/1 -> SEA Kalman Filter2/3
  Selector26/1 -> Mux10/2
  Selector27/1 -> Mux10/3
  [LoadVelocity] -> Selector27/1
  [MotorVelocity] -> Selector26/1
  Mux10/1 -> Selector28/1
  [LoadAbsolute] -> Selector25/1
  [MotorIncremental] -> Selector24/1
  [MotorAbsolute] -> Selector23/1
  Selector23/1 -> Mux9/1
  Selector24/1 -> Mux9/2
  Selector25/1 -> Mux9/3
  [TrunkTorque] -> Selector22/1
  [SpringTorque] -> Selector20/1
  Selector22/1 -> Mux8/3
  Selector20/1 -> Mux8/2
  [RotorTorque] -> Selector21/1
  Selector21/1 -> Mux8/1
  Mux9/1 -> SEA Kalman Filter2/2, Mux10/1
  SEA Kalman Filter1/1 -> Demux2/1
  [Q2] -> SEA Kalman Filter1/6
  [R2] -> SEA Kalman Filter1/7
  Constant4/1 -> SEA Kalman Filter1/5
  Constant1/1 -> SEA Kalman Filter1/4
  Selector5/1 -> SEA Kalman Filter1/3
  Selector18/1 -> Mux7/2
  Selector19/1 -> Mux7/3
  [LoadVelocity] -> Selector19/1
  [MotorVelocity] -> Selector18/1
  Mux7/1 -> Selector5/1
  [LoadAbsolute] -> Selector17/1
  [MotorIncremental] -> Selector4/1
  [MotorAbsolute] -> Selector3/1
  Selector3/1 -> Mux6/1
  Selector4/1 -> Mux6/2
  Selector17/1 -> Mux6/3
  [TrunkTorque] -> Selector2/1
  [SpringTorque] -> Selector1/1
  Selector2/1 -> Mux5/3
  Selector1/1 -> Mux5/2
  [RotorTorque] -> Selector16/1
  Selector16/1 -> Mux5/1
  Mux6/1 -> Mux7/1, SEA Kalman Filter1/2
  Mux5/1 -> SEA Kalman Filter1/1
  Covariance Estimates/8(R4) -> [R4]
  Covariance Estimates/6(R3) -> [R3]
  Covariance Estimates/4(R2) -> [R2]
  Covariance Estimates/2(R1) -> [R1]
  Covariance Estimates/7(Q4) -> [Q4]
  Covariance Estimates/5(Q3) -> [Q3]
  Covariance Estimates/3(Q2) -> [Q2]
  Covariance Estimates/1(Q1) -> [Q1]
  [SpringTorque] -> Covariance Estimates/1(spring_torque)
  Mux4/1 -> Filtered Motor Positions [rad] x4/1
  SEA Kalman Filter/1 -> Demux1/1
  [Q1] -> SEA Kalman Filter/6
  [R1] -> SEA Kalman Filter/7
  Constant3/1 -> SEA Kalman Filter/5
  Constant2/1 -> SEA Kalman Filter/4
  Selector15/1 -> SEA Kalman Filter/3
  Selector13/1 -> Mux3/2
  Selector14/1 -> Mux3/3
  [LoadVelocity] -> Selector14/1
  [MotorVelocity] -> Selector13/1
  Mux3/1 -> Selector15/1
  "Load Velocity, Initial [rad/s] x4"/1 -> [LoadVelocity]
  "Motor Velocity, Initial [rad/s] x4"/1 -> [MotorVelocity]
  [LoadAbsolute] -> Selector11/1
  [MotorIncremental] -> Selector10/1
  [MotorAbsolute] -> Selector9/1
  Selector9/1 -> Mux2/1
  Selector10/1 -> Mux2/2
  Selector11/1 -> Mux2/3
  [TrunkTorque] -> Selector8/1
  [SpringTorque] -> Selector7/1
  Selector8/1 -> Mux1/3
  Selector7/1 -> Mux1/2
  [RotorTorque] -> Selector6/1
  Selector6/1 -> Mux1/1
  Mux2/1 -> SEA Kalman Filter/2, Mux3/1
  Mux1/1 -> SEA Kalman Filter/1
  External Trunk Torque [Nm] x4/1 -> [TrunkTorque]
  "Load Position, Absolute [rad] x4"/1 -> [LoadAbsolute]
  "Motor Position, Absolute [rad] x4"/1 -> [MotorAbsolute]
  Rotor Torque [Nm] x4/1 -> [RotorTorque]
  Spring Torque [Nm] x4/1 -> [SpringTorque]
  "Motor Position, Incremental [rad] x4"/1 -> [MotorIncremental]
  Mux8/1 -> SEA Kalman Filter2/1

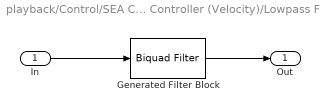
== system playback/Control/SEA Control/SEA Controller (Velocity)/Lowpass Filter ==
  In : Inport
  Generated Filter Block : dsparch4/Biquad Filter  Tag=BlockMethodSubSystem  IIRFiltStruct=Direct form II  CoeffSource=Specify via dialog  BiQuadCoeffs=[0.60519205517212682 -0.19552086280129813 0.60519205517212682 1 -1.2952421271021082 0.49678687396485205]  a0Flag=Warning  IC=0  ICnum=0  ICden=0  denAccumFracLength=30  denProdOutputFracLength=30  secondMemoryFracLength=15  roundingMode=Floor  overflowMode=off  ScaleValues=[0.19859300979781833;1]  optimizeScaleValues=off  ScaleValueMode=Specify via input port (g)  scaleValueFracLength=14  FilterSource=Specify via dialog  FilterObject=BQF
  Out : Outport
  wires:
  In/1 -> Generated Filter Block/1
  Generated Filter Block/1 -> Out/1

== matlab function playback/Control/SEA Control/SEA Kalman Filter (swing)/Covariance Estimates ==
  data: spring_torque input; absolute_motor input; absolute_load input; Q1 output; R1 output; Q2 output; R2 output; R_kalman_absolute_normal parameter; R_kalman_absolute_fail parameter; R_kalman_incremental_unloaded parameter; R_kalman_incremental_loaded parameter; kalman_load_to_deflect_transmission parameter; Q3 output; R3 output; Q4 output; R4 output; Q_kalman_spring_torque parameter; Q_kalman_rotor_torque parameter; Q_kalman_trunk_torque parameter; sample_time parameter
function [Q1, R1, Q2, R2, Q3, R3, Q4, R4] = covariance( spring_torque, absolute_motor, absolute_load, R_kalman_absolute_normal, R_kalman_absolute_fail, R_kalman_incremental_unloaded, R_kalman_incremental_loaded, kalman_load_to_deflect_transmission, Q_kalman_spring_torque, Q_kalman_rotor_torque, Q_kalman_trunk_torque, sample_time)

    % Initialize persistent absolute measurement variables
    persistent previous_absolute_gear previous_absolute_load
    if isempty(previous_absolute_gear)
        previous_absolute_gear = absolute_motor;
    end
    if isempty(previous_absolute_load)
        previous_absolute_load = absolute_load;
    end
    
    % Measurement covariance
    R_absolute_motor = ones(4,1)*R_kalman_absolute_normal;
    R_absolute_load = ones(4,1)*R_kalman_absolute_normal;
    dropped_out = previous_absolute_gear == absolute_motor;
   % R_absolute_motor(dropped_out) = R_kalman_absolute_fail;
    dropped_out = previous_absolute_load == absolute_load;
   % R_absolute_load(dropped_out) = R_kalman_absolute_fail;
    R_incremental_scale = min(abs(spring_torque)/kalman_load_to_deflect_transmission, 1);
    R_incremental = R_incremental_scale*R_kalman_incremental_loaded + (1-R_incremental_scale)*R_kalman_incremental_unloaded;
    R1 = diag([R_absolute_motor(1), R_incremental(1), R_absolute_load(1)])/sample_time;
    R2 = diag([R_absolute_motor(2), R_incremental(2), R_absolute_load(2)])/sample_time;
    R3 = diag([R_absolute_motor(3), R_incremental(3), R_absolute_load(3)])/sample_time;
    R4 = diag([R_absolute_motor(4), R_incremental(4), R_absolute_load(4)])/sample_time;
    
    % Process noise covariance
    Q_spring_torque = ones(4,1)*Q_kalman_spring_torque; % + k_sea_low.^2.*(state_uncertainty + R_kalman_absolute_normal)
    Q1 = diag([Q_kalman_rotor_torque, Q_spring_torque(1), Q_kalman_trunk_torque]);
    Q2 = diag([Q_kalman_rotor_torque, Q_spring_torque(2), Q_kalman_trunk_torque]);
    Q3 = diag([Q_kalman_rotor_torque, Q_spring_torque(3), Q_kalman_trunk_torque]);
    Q4 = diag([Q_kalman_rotor_torque, Q_spring_torque(4), Q_kalman_trunk_torque]);

    previous_absolute_gear = absolute_motor;
    previous_absolute_load = absolute_load;
end

== matlab function playback/Control/SEA Control/SEA Controller (Velocity)/Nonlinear Spring Force ==
  data: deflections input; tau_sea output
function tau_sea   = SeaSpringForce( deflections )
    tau_sea = SeaSpringForce( deflections );
end
